simulink model "openclosedloopwithdisturbance"  (R2021a)
settings: Solver=VariableStepAuto  StartTime=0.0  StopTime=10.0  RelTol=1e-3
settings Model: Creator=user  LastModifiedBy=user

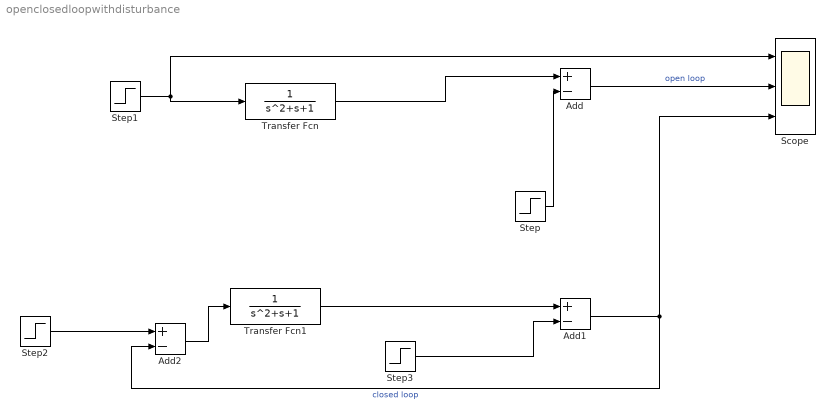
== system openclosedloopwithdisturbance ==
  Add : Sum  Inputs=+-
  Add1 : Sum  Inputs=+-
  Add2 : Sum  Inputs=+-
  Scope : Scope  NumInputPorts=3
  Step : Step  Time=4  After=0.4  SampleTime=0
  Step1 : Step  SampleTime=0
  Step2 : Step  SampleTime=0
  Step3 : Step  Time=4  After=0.4  SampleTime=0
  Transfer Fcn : TransferFcn  Denominator=[1 1 1]
  Transfer Fcn1 : TransferFcn  Denominator=[1 1 1]
  wires:
  Step1/1 -> Scope/1, Transfer Fcn/1
  Transfer Fcn/1 -> Add/1
  Step/1 -> Add/2
  Add/1 -> Scope/2  "open loop"
  Transfer Fcn1/1 -> Add1/1
  Step3/1 -> Add1/2
  Step2/1 -> Add2/1
  Add2/1 -> Transfer Fcn1/1
  Add1/1 -> Scope/3, Add2/2  "closed loop"
